simulink model "plc_diagram"  (R2026a)
settings: Solver=ode15s  StopTime=15.0  MaxStep=0.3
settings Model: Creator=zoyab  LastModifiedBy=zoyab

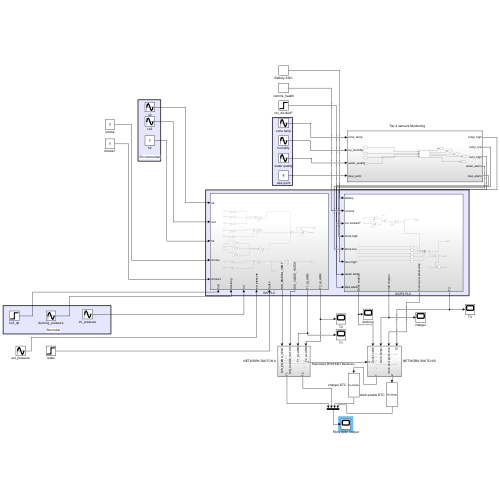
[thumbnail: Simulink's stored preview of the top-level diagram]
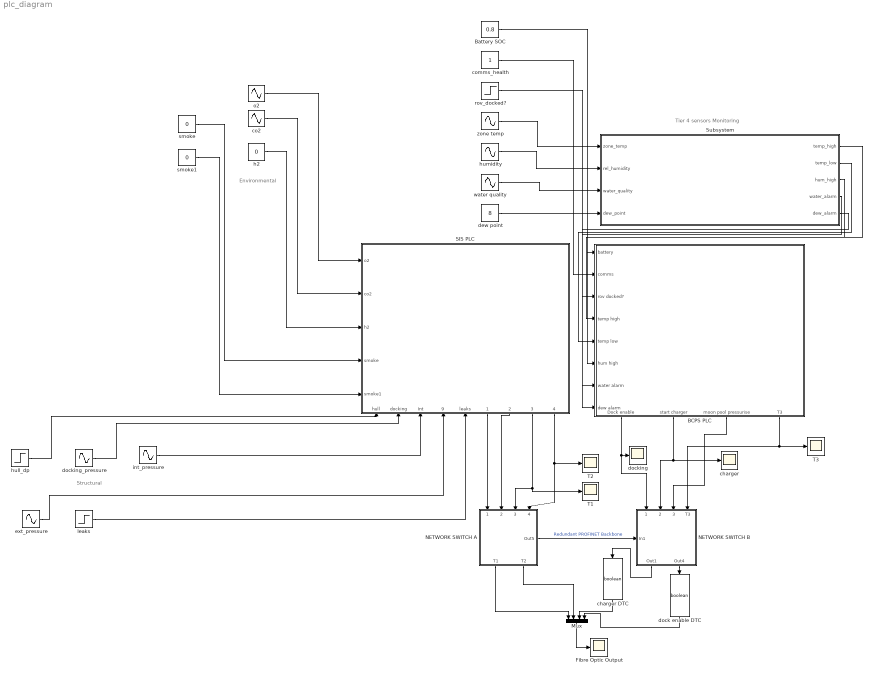
== system plc_diagram ==
  note: Tier 4 sensors Monitoring
  note: Environmental
  note: Structural
  BCPS PLC : Subsystem
      settings: PortSchema="{\"entries\":[{\"content\":{\"sides\":[{\"content\":{\"connectorIds\":[\"In1\",\"In2\",\"In3\",\"In4\",\"In5\",\"In6\",\"In7\",\"In8\"]},\"type\":\"ConnectorPlacement.EquallySpacedRectSide\",\"uuid\":\"fafd5387-af76-4b64-82a4-bdebbe500840\"},{\"content\":{\"side\":\"RIGHT\"},\"type\":\"ConnectorPlacement.EquallySpacedRectSide\",\"uuid\":\"d9ebb9fa-a634-460a-b1d6-d44ee4ae1f2b\"},{\"content\":{\"side\":\"TOP\"},\"type\":\"ConnectorPlacement.EquallySpacedRectSide\",\"uuid\":\"b37c090d-f37e-45b2-8247-c9e459ca9a95\"},{\"content\":{\"connectorIds\":[\"Out1\",\"Out2\",\"Out3\",\"Out4\"],\"side\":\"BOTTOM\"},\"type\":\"ConnectorPlacement.EquallySpacedRectSide\",\"uuid\":\"f2869c88-519b-4802-8a7f-76a17c6323f5\"}]},\"type\":\"ConnectorPlacement.EquallySpacedConnector\",\"uuid\":\"1bec988e-95c9-4b4b-ad53-675dcb77e0ad\"}],\"packageUris\":[\"http://schema.mathworks.com/mf0/Connector/R2020b\"],\"version\":\"1.0\"}"
  Battery SOC : Constant  Value=0.8
  Fibre Optic Output : Scope
      settings: ActiveDisplayYMinimum=-8.8498710065528812  ActiveDisplayYMaximum=8.6192917530981141  DataLoggingVariableName=ScopeData6
  Mux : Mux
  NETWORK SWITCH A : Subsystem
      settings: PortSchema="{\"entries\":[{\"content\":{\"sides\":[{\"content\":{\"connectorIds\":[\"In1\",\"In2\",\"In3\",\"In4\"]},\"type\":\"ConnectorPlacement.EquallySpacedRectSide\",\"uuid\":\"95487d7c-fcff-4633-a60c-20359c103332\"},{\"content\":{\"connectorIds\":[\"Out1\",\"Out2\"],\"side\":\"RIGHT\"},\"type\":\"ConnectorPlacement.EquallySpacedRectSide\",\"uuid\":\"d14fabc7-d34d-4620-ba8d-af8f2c860048\"},{\"content\":{\"side\":\"TOP\"},\"type\":\"ConnectorPlacement.EquallySpacedRectSide\",\"uuid\":\"28751fd4-9240-4734-925c-6db0db9fed3c\"},{\"content\":{\"connectorIds\":[\"Out3\"],\"side\":\"BOTTOM\"},\"type\":\"ConnectorPlacement.EquallySpacedRectSide\",\"uuid\":\"716f5af4-56a6-450b-ac5b-994213927138\"}]},\"type\":\"ConnectorPlacement.EquallySpacedConnector\",\"uuid\":\"4c4809b0-8d8f-4bbb-8d5b-8137454220da\"}],\"packageUris\":[\"http://schema.mathworks.com/mf0/Connector/R2020b\"],\"version\":\"1.0\"}"
  NETWORK SWITCH B : Subsystem
      settings: PortSchema="{\"entries\":[{\"content\":{\"sides\":[{\"content\":{\"connectorIds\":[\"In1\",\"In2\",\"In3\",\"In4\"]},\"type\":\"ConnectorPlacement.EquallySpacedRectSide\",\"uuid\":\"b74aa3e2-82d3-4b7a-864c-cdd6d937eed7\"},{\"content\":{\"connectorIds\":[\"Out1\",\"Out2\"],\"side\":\"RIGHT\"},\"type\":\"ConnectorPlacement.EquallySpacedRectSide\",\"uuid\":\"e1ee4ad3-d048-4597-aa4a-202a008bbd3d\"},{\"content\":{\"connectorIds\":[\"In5\"],\"side\":\"TOP\"},\"type\":\"ConnectorPlacement.EquallySpacedRectSide\",\"uuid\":\"47b64970-9100-4474-9486-ab2a98e76139\"}]},\"type\":\"ConnectorPlacement.EquallySpacedConnector\",\"uuid\":\"4bdf1fd7-8289-4a28-9e62-10058d5e0580\"}],\"packageUris\":[\"http://schema.mathworks.com/mf0/Connector/R2020b\"],\"version\":\"1.0\"}"
  SIS PLC : Subsystem
      settings: PortSchema="{\"entries\":[{\"content\":{\"sides\":[{\"content\":{\"connectorIds\":[\"In1\",\"In2\",\"In3\",\"In4\",\"In5\"]},\"type\":\"ConnectorPlacement.EquallySpacedRectSide\",\"uuid\":\"34d54887-c06f-4d89-a29c-e3e22c49bba5\"},{\"content\":{\"side\":\"RIGHT\"},\"type\":\"ConnectorPlacement.EquallySpacedRectSide\",\"uuid\":\"b1c8ee0c-fdc6-4d95-b4f3-b112114acf63\"},{\"content\":{\"side\":\"TOP\"},\"type\":\"ConnectorPlacement.EquallySpacedRectSide\",\"uuid\":\"5434bdaf-e38b-4bdb-b2da-0f69e16c54f3\"},{\"content\":{\"connectorIds\":[\"In6\",\"In7\",\"In8\",\"In9\",\"In10\",\"Out1\",\"Out2\",\"Out3\",\"Out4\"],\"side\":\"BOTTOM\"},\"type\":\"ConnectorPlacement.EquallySpacedRectSide\",\"uuid\":\"a4ad84cd-e496-4637-b969-ba70c37ca6b3\"}]},\"type\":\"ConnectorPlacement.EquallySpacedConnector\",\"uuid\":\"3de58dc7-e406-4fc9-ae08-7f02da552cf7\"}],\"packageUris\":[\"http://schema.mathworks.com/mf0/Connector/R2020b\"],\"version\":\"1.0\"}"
  Subsystem : Subsystem
  T1 : Scope
      settings: ActiveDisplayYMinimum=-8.0125424974215  ActiveDisplayYMaximum=4.0488806035737017
  T2 : Scope
      settings: ActiveDisplayYMinimum=-15.890470997739884  ActiveDisplayYMaximum=15.769505077927985
  T3 : Scope
      settings: ActiveDisplayYMinimum=0.99832474352108258  ActiveDisplayYMaximum=1.0013226015395793  DataLoggingVariableName=ScopeData2
  charger : Scope
      settings: ActiveDisplayYMinimum=-0.77152839301733311  ActiveDisplayYMaximum=2.1519843571843538  DataLoggingVariableName=ScopeData4
  charger DTC : DataTypeConversion  OutDataTypeStr=boolean  SaturateOnIntegerOverflow=off  RndMeth=Floor
  co2 : Sin  Amplitude=50  Bias=450  Frequency=0.08  SampleTime=0
  comms_health : Constant
  dew point : Constant  Value=8
  dock enable DTC : DataTypeConversion  OutDataTypeStr=boolean  SaturateOnIntegerOverflow=off  RndMeth=Floor
  docking : Scope
      settings: ActiveDisplayYMinimum=0.61209772467556334  ActiveDisplayYMaximum=1.5821428151295645  DataLoggingVariableName=ScopeData3
  docking_pressure : Sin  Amplitude=0.3  Bias=11  Frequency=0.05  SampleTime=0
  ext_pressure : Sin  Amplitude=0.3  Bias=11  Frequency=0.05  SampleTime=0
  h2 : Constant  Value=0
  hull_dp : Step  Time=7  FinalValue=1.5  SampleTime=0
  humidity : Sin  Amplitude=5  Bias=45  Frequency=0.015  SampleTime=0
  int_pressure : Sin  Amplitude=0.1  Bias=11  Frequency=0.04  SampleTime=0
  leaks : Step  Time=7  SampleTime=0
  o2 : Sin  Amplitude=0.5  Bias=21  Frequency=0.1  SampleTime=0
  rov_docked? : Step  SampleTime=0
  smoke : Constant  Value=0
  smoke1 : Constant  Value=0
  water quality : Sin  Amplitude=5  Bias=25  Phase=0.01  SampleTime=0
  zone temp : Sin  Bias=21  Frequency=0.02  SampleTime=0
  wires:
  o2/1 -> SIS PLC/1(o2)
  co2/1 -> SIS PLC/2(co2)
  h2/1 -> SIS PLC/3(h2)
  smoke/1 -> SIS PLC/4(smoke)
  smoke1/1 -> SIS PLC/5(smoke1)
  hull_dp/1 -> SIS PLC/6(hull)
  int_pressure/1 -> SIS PLC/8(Int)
  docking_pressure/1 -> SIS PLC/7(docking)
  ext_pressure/1 -> SIS PLC/9(ext pressure)
  leaks/1 -> SIS PLC/10(leaks)
  dew point/1 -> Subsystem/4(dew_point)
  humidity/1 -> Subsystem/2(rel_humidity)
  water quality/1 -> Subsystem/3(water_quality)
  zone temp/1 -> Subsystem/1(zone_temp)
  rov_docked?/1 -> BCPS PLC/3(rov docked?)
  comms_health/1 -> BCPS PLC/2(comms)
  Battery SOC/1 -> BCPS PLC/1(battery)
  SIS PLC/1(SIS_EMERG_VENT) -> NETWORK SWITCH A/1(SIS_EMERG_VENT)
  SIS PLC/2(SIS_CLOSE_HATCH) -> NETWORK SWITCH A/2(SIS_CLOSE_HATCH)
  SIS PLC/3(T1_ALARM) -> T1/1, NETWORK SWITCH A/3(T1_ALARM)
  SIS PLC/4(T2_ALARM) -> T2/1, NETWORK SWITCH A/4(T2_ALARM)
  BCPS PLC/2(start charger) -> NETWORK SWITCH B/2(start charger), charger/1
  BCPS PLC/3(moon pool pressurise) -> NETWORK SWITCH B/3(moon pool pressurise)
  BCPS PLC/4(T3) -> T3/1, NETWORK SWITCH B/4(T3)
  NETWORK SWITCH A/3(Out5) -> NETWORK SWITCH B/5(In1)  "Redundant PROFINET Backbone"
  BCPS PLC/1(Dock enable) -> docking/1, NETWORK SWITCH B/1(Dock enable)
  NETWORK SWITCH A/1(T1) -> Mux/1
  NETWORK SWITCH A/2(T2) -> Mux/2
  Mux/1 -> Fibre Optic Output/1
  charger DTC/1 -> Mux/3
  NETWORK SWITCH B/1(Out1) -> charger DTC/1
  NETWORK SWITCH B/2(Out4) -> dock enable DTC/1
  dock enable DTC/1 -> Mux/4
  Subsystem/1(temp_high) -> BCPS PLC/4(temp high)
  Subsystem/2(temp_low) -> BCPS PLC/5(temp low)
  Subsystem/3(hum_high) -> BCPS PLC/6(hum high)
  Subsystem/4(water_alarm) -> BCPS PLC/7(water alarm)
  Subsystem/5(dew_alarm) -> BCPS PLC/8(dew alarm)

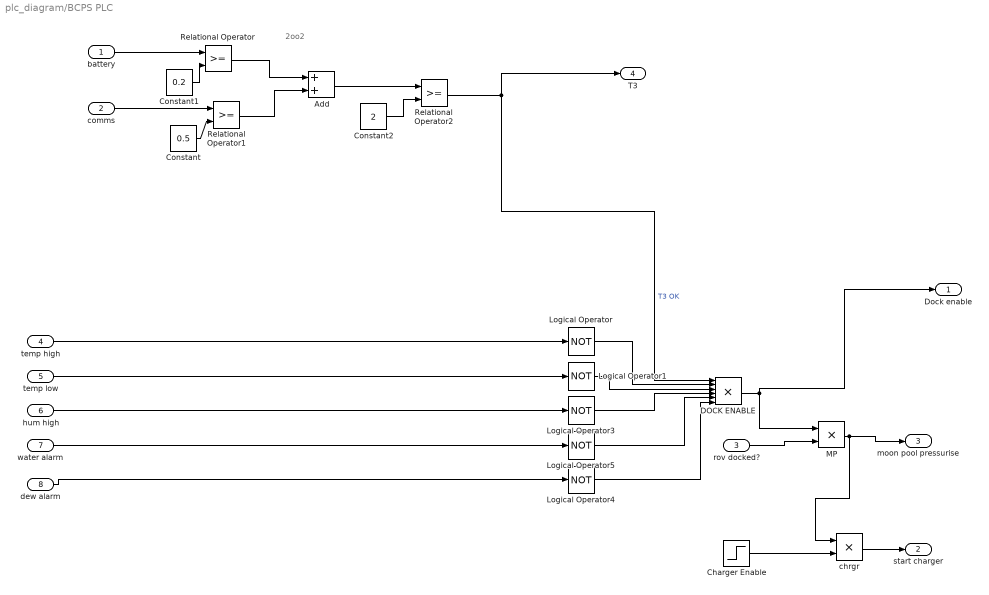
== system plc_diagram/BCPS PLC ==
  note: 2oo2
  battery : Inport
  comms : Inport  Port=2
  rov docked? : Inport  Port=3
  temp high : Inport  Port=4
  temp low : Inport  Port=5
  hum high : Inport  Port=6
  water alarm : Inport  Port=7
  dew alarm : Inport  Port=8
  Add : Sum
  Charger Enable : Step  Time=10  SampleTime=0
  Constant : Constant  Value=0.5
  Constant1 : Constant  Value=0.2
  Constant2 : Constant  Value=2
  DOCK ENABLE : Product  Inputs=6
  Logical Operator{,1,3..5} (5 alike) : Logic  Operator=NOT  AllPortsSameDT=off  OutDataTypeStr=boolean
  MP : Product
  Relational Operator : RelationalOperator  OutDataTypeStr=boolean  RndMeth=Simplest  InputSameDT=off
  Relational Operator1 : RelationalOperator  OutDataTypeStr=boolean  RndMeth=Simplest  InputSameDT=off
  Relational Operator2 : RelationalOperator  OutDataTypeStr=boolean  RndMeth=Simplest  InputSameDT=off
  chrgr : Product
  Dock enable : Outport
  start charger : Outport  Port=2
  moon pool pressurise : Outport  Port=3
  T3 : Outport  Port=4
  wires:
  Constant/1 -> Relational Operator1/2
  Constant1/1 -> Relational Operator/2
  Relational Operator/1 -> Add/1
  Relational Operator1/1 -> Add/2
  Add/1 -> Relational Operator2/1
  Constant2/1 -> Relational Operator2/2
  Relational Operator2/1 -> DOCK ENABLE/1, T3/1  "T3 OK"
  Logical Operator/1 -> DOCK ENABLE/2
  Logical Operator1/1 -> DOCK ENABLE/3
  Logical Operator3/1 -> DOCK ENABLE/4
  Logical Operator5/1 -> DOCK ENABLE/5
  Logical Operator4/1 -> DOCK ENABLE/6
  DOCK ENABLE/1 -> Dock enable/1, MP/1
  rov docked?/1 -> MP/2
  MP/1 -> chrgr/1, moon pool pressurise/1
  Charger Enable/1 -> chrgr/2
  chrgr/1 -> start charger/1
  temp high/1 -> Logical Operator/1
  temp low/1 -> Logical Operator1/1
  dew alarm/1 -> Logical Operator4/1
  water alarm/1 -> Logical Operator5/1
  hum high/1 -> Logical Operator3/1
  battery/1 -> Relational Operator/1
  comms/1 -> Relational Operator1/1

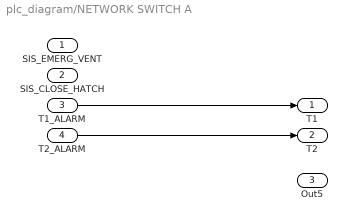
== system plc_diagram/NETWORK SWITCH A ==
  SIS_EMERG_VENT : Inport
  SIS_CLOSE_HATCH : Inport  Port=2
  T1_ALARM : Inport  Port=3
  T2_ALARM : Inport  Port=4
  T1 : Outport
  T2 : Outport  Port=2
  Out5 : Outport  Port=3
  wires:
  T1_ALARM/1 -> T1/1
  T2_ALARM/1 -> T2/1

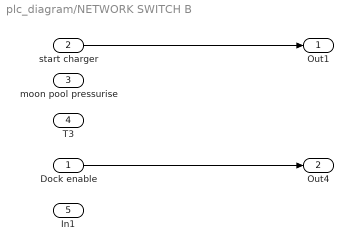
== system plc_diagram/NETWORK SWITCH B ==
  Dock enable : Inport
  start charger : Inport  Port=2
  moon pool pressurise : Inport  Port=3
  T3 : Inport  Port=4
  In1 : Inport  Port=5
  Out1 : Outport
  Out4 : Outport  Port=2
  wires:
  start charger/1 -> Out1/1
  Dock enable/1 -> Out4/1

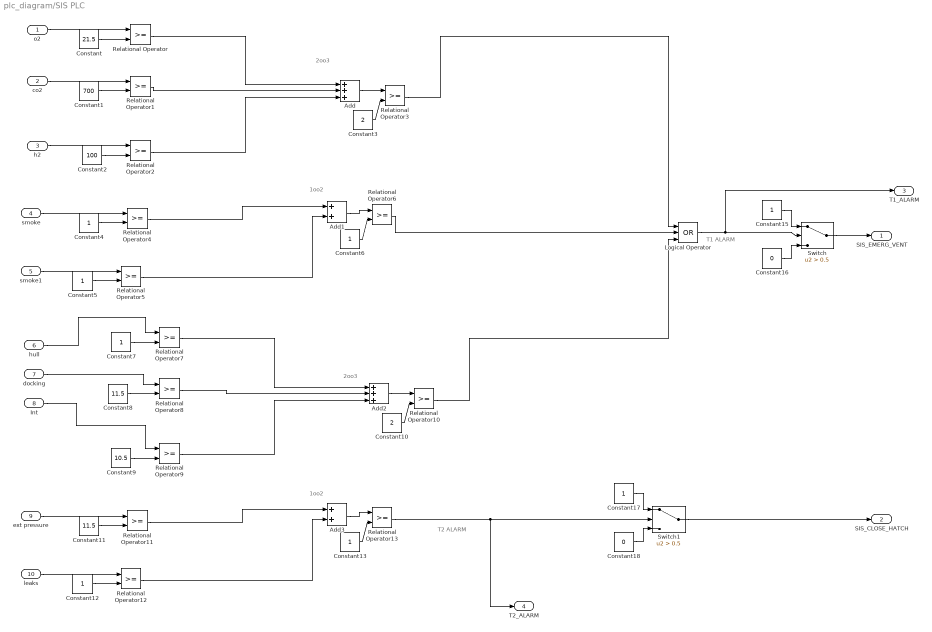
== system plc_diagram/SIS PLC ==
  note: 2oo3
  note: 2oo3
  note: 1oo2
  note: 1oo2
  note: T1 ALARM
  note: T2 ALARM
  o2 : Inport
  co2 : Inport  Port=2
  h2 : Inport  Port=3
  smoke : Inport  Port=4
  smoke1 : Inport  Port=5
  hull : Inport  Port=6
  docking : Inport  Port=7
  Int : Inport  Port=8
  ext pressure : Inport  Port=9
  leaks : Inport  Port=10
  Add : Sum  Inputs=+++
  Add1 : Sum
  Add2 : Sum  Inputs=+++
  Add3 : Sum
  Constant : Constant  Value=21.5
  Constant1 : Constant  Value=700
  Constant10 : Constant  Value=2
  Constant11 : Constant  Value=11.5
  Constant{4..7,12..13,15,17} (8 alike) : Constant
  Constant16 : Constant  Value=0
  Constant18 : Constant  Value=0
  Constant2 : Constant  Value=100
  Constant3 : Constant  Value=2
  Constant8 : Constant  Value=11.5
  Constant9 : Constant  Value=10.5
  Logical Operator : Logic  Operator=OR  Inputs=3  AllPortsSameDT=off  OutDataTypeStr=boolean
  Relational Operator{,1..13} (14 alike) : RelationalOperator  OutDataTypeStr=boolean  RndMeth=Simplest  InputSameDT=off
  Switch : Switch  Criteria=u2 > Threshold  Threshold=0.5  SaturateOnIntegerOverflow=off  InputSameDT=off
  Switch1 : Switch  Criteria=u2 > Threshold  Threshold=0.5  SaturateOnIntegerOverflow=off  InputSameDT=off
  SIS_EMERG_VENT : Outport
  SIS_CLOSE_HATCH : Outport  Port=2
  T1_ALARM : Outport  Port=3
  T2_ALARM : Outport  Port=4
  wires:
  o2/1 -> Relational Operator/1
  Constant/1 -> Relational Operator/2
  co2/1 -> Relational Operator1/1
  Constant1/1 -> Relational Operator1/2
  h2/1 -> Relational Operator2/1
  Constant2/1 -> Relational Operator2/2
  Relational Operator/1 -> Add/1
  Relational Operator1/1 -> Add/2
  Relational Operator2/1 -> Add/3
  Add/1 -> Relational Operator3/1
  Constant3/1 -> Relational Operator3/2
  Relational Operator3/1 -> Logical Operator/1
  Constant4/1 -> Relational Operator4/2
  Relational Operator4/1 -> Add1/1
  smoke/1 -> Relational Operator4/1
  Constant5/1 -> Relational Operator5/2
  Relational Operator5/1 -> Add1/2
  smoke1/1 -> Relational Operator5/1
  Relational Operator6/1 -> Logical Operator/2
  Add1/1 -> Relational Operator6/1
  Constant6/1 -> Relational Operator6/2
  Relational Operator10/1 -> Logical Operator/3
  hull/1 -> Relational Operator7/1
  Constant7/1 -> Relational Operator7/2
  Constant10/1 -> Relational Operator10/2
  Relational Operator8/1 -> Add2/2
  Relational Operator7/1 -> Add2/1
  Constant9/1 -> Relational Operator9/2
  Constant8/1 -> Relational Operator8/2
  docking/1 -> Relational Operator8/1
  Add2/1 -> Relational Operator10/1
  Relational Operator9/1 -> Add2/3
  Int/1 -> Relational Operator9/1
  Constant11/1 -> Relational Operator11/2
  Relational Operator12/1 -> Add3/2
  Add3/1 -> Relational Operator13/1
  Constant13/1 -> Relational Operator13/2
  Relational Operator11/1 -> Add3/1
  Constant12/1 -> Relational Operator12/2
  ext pressure/1 -> Relational Operator11/1
  leaks/1 -> Relational Operator12/1
  Switch/1 -> SIS_EMERG_VENT/1
  Logical Operator/1 -> Switch/2, T1_ALARM/1
  Constant15/1 -> Switch/1
  Constant16/1 -> Switch/3
  Constant17/1 -> Switch1/1
  Relational Operator13/1 -> T2_ALARM/1, Switch1/2
  Constant18/1 -> Switch1/3
  Switch1/1 -> SIS_CLOSE_HATCH/1

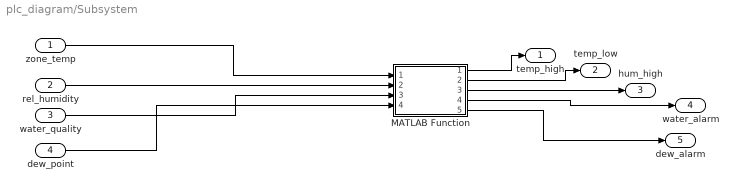
== system plc_diagram/Subsystem ==
  zone_temp : Inport
  rel_humidity : Inport  Port=2
  water_quality : Inport  Port=3
  dew_point : Inport  Port=4
  MATLAB Function : MATLAB Function  TreatAsAtomicUnit=on
  temp_high : Outport
  temp_low : Outport  Port=2
  hum_high : Outport  Port=3
  water_alarm : Outport  Port=4
  dew_alarm : Outport  Port=5
  wires:
  water_quality/1 -> MATLAB Function/3(water_quality)
  rel_humidity/1 -> MATLAB Function/2(rel_humidity)
  zone_temp/1 -> MATLAB Function/1(zone_temp)
  dew_point/1 -> MATLAB Function/4(dew_point)
  MATLAB Function/1(temp_high) -> temp_high/1
  MATLAB Function/2(temp_low) -> temp_low/1
  MATLAB Function/3(hum_high) -> hum_high/1
  MATLAB Function/4(water_alarm) -> water_alarm/1
  MATLAB Function/5(dew_alarm) -> dew_alarm/1

== matlab function plc_diagram/Subsystem/MATLAB Function ==
  data: zone_temp input; temp_high output; rel_humidity input; water_quality input; dew_point input; temp_low output; hum_high output; water_alarm output; dew_alarm output
function [temp_high, temp_low, hum_high, water_alarm, dew_alarm] = env_monitor(zone_temp, rel_humidity, water_quality, dew_point)
% Zone temperature alarms (LIFE SUPPORT spec: 18-24°C)
% Humidity alarm (LIFE SUPPORT spec: 30-60% RH)
% Water quality alarm (LIFE SUPPORT spec: <=50 CFU/mL)
% Dew point alarm (LIFE SUPPORT spec: <12°C)
temp_high = double(zone_temp >= 24);
temp_low  = double(zone_temp <= 18);
hum_high  = double(rel_humidity >= 60);
water_alarm = double(water_quality >= 50);
dew_alarm = double(dew_point >= 12);
